simulink model "reaction_wheel_controller"  (R2024b)
settings: Solver=VariableStepAuto  StartTime=0.0  StopTime=10.0  RelTol=1e-3
undefined symbols (not defined in the file): Kd, Kp
settings Model: Creator=conno  LastModifiedBy=conno

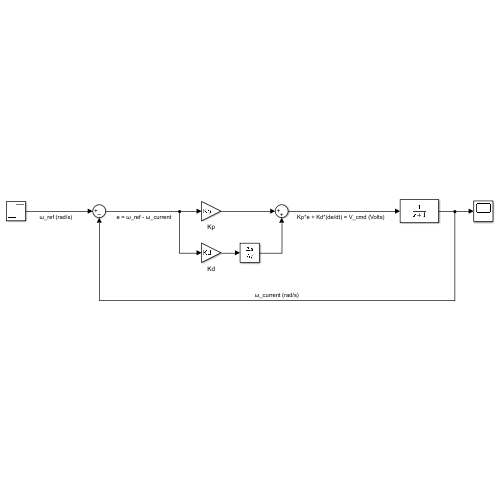
[thumbnail: Simulink's stored preview of the top-level diagram]
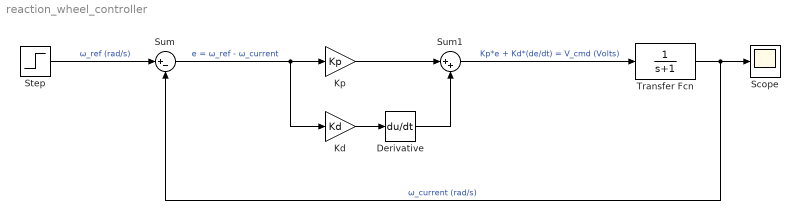
== system reaction_wheel_controller ==
  Derivative : Derivative
  Kd : Gain  Gain=Kd
  Kp : Gain  Gain=Kp
  Scope : Scope
  Step : Step  SampleTime=0
  Sum : Sum  Inputs=|+-
  Sum1 : Sum  Inputs=|++
  Transfer Fcn : TransferFcn  Denominator=[1 1]
  wires:
  Sum1/1 -> Transfer Fcn/1  "Kp*e + Kd*(de/dt) = V_cmd (Volts)"
  Step/1 -> Sum/1  "ω_ref (rad/s)"
  Sum/1 -> Kd/1, Kp/1  "e = ω_ref - ω_current"
  Kd/1 -> Derivative/1
  Kp/1 -> Sum1/1
  Transfer Fcn/1 -> Sum/2, Scope/1  "ω_current (rad/s)"
  Derivative/1 -> Sum1/2
